simulink model "Project_SC"  (R2022a)
settings: Solver=FixedStepAuto  StartTime=0.0  StopTime=t_stop*5  FixedStep=t_step  EnableMultiTasking=on
values from neighbouring files (symbols this model uses):
  Ib = 1723*sqrt(2)    [analyticalStuff.m]
  J = p/2*Pb*M/(wmb^2)    (= 2380.03460376)    [analyticalStuff.m]
  p = 6    [analyticalStuff.m]
  Rr = 1.39e-3    (= 0.00139)    [analyticalStuff.m]
  Rs = 1.343e-3    (= 0.001343)    [analyticalStuff.m]
  Tb = 13.944e3    (= 13944)    [analyticalStuff.m]    (also in plotTorqueSpeedCurve.m)
  Tload = data.Tload    [plotTorqueSpeedCurve.m]    (also in torqueSpeedCurveData.mat = [-69720 -66874.2857143 -64028.5714286 -61182.8571429 -58337.)
  Vb = 331.98*sqrt(2)    [analyticalStuff.m]
  wb = 2*pi*fb    (= 314.159265359)    [analyticalStuff.m]
  we = 2*pi*fb    (= 314.159265359)    [analyticalStuff.m]
  Xlr = Llr*we    (= 0.0156451314149)    [analyticalStuff.m]
  Xls = Lls*we    (= 0.0327982273035)    [analyticalStuff.m]
  Xmstar = 1/(1/Xls+1/Xm+1/Xlr)    (= 0.0103944378454)    [analyticalStuff.m]
undefined symbols (not defined in the file or in its folder): fdr0, fds0, fqr0, fqs0, k, t_fault, wrotor_init
settings Model: Creator=kavita  LastModifiedBy=cakal
settings SolverCC: MaxConsecutiveZCs=1  ZeroCrossAlgorithm=Adaptive  AlgebraicLoopSolver=TrustRegion
settings DataIOCC: LimitDataPoints=on  SaveFormat=Array  SignalLoggingSaveFormat=ModelDataLogs  ReturnWorkspaceOutputs=off
settings OptimizationCC: ExpressionDepthLimit=2147483647  LifeSpan=inf
settings DebuggingCC: UnderspecifiedInitializationDetection=Classic  MergeDetectMultiDrivingBlocksExec=none  SolverPrmCheckMsg=warning  FcnCallInpInsideContextMsg=warning  UnconnectedInputMsg=warning  UnconnectedOutputMsg=warning  UnconnectedLineMsg=warning  StateNameClashWarn=warning  SFUnexpectedBacktrackingDiag=warning  SFNoUnconditionalDefaultTransitionDiag=warning  SFExecutionAtInitializationDiag=none  SFMachineParentedDataDiag=warning  ArithmeticOperatorsInVariantConditions=warning
settings HardwareCC: ProdBitPerPointer=32  ProdBitPerSizeT=32  ProdBitPerPtrDiffT=32  ProdLargestAtomicFloat=None  ProdIntDivRoundTo=Undefined  ProdEndianess=Unspecified  ProdWordSize=32  ProdHWDeviceType=32-bit Generic
settings ModelReferenceCC: PropagateSignalLabelsOutOfModel=off
settings SFSimCC: SimUseLocalCustomCode=off  CustomCodeUndefinedFunction=UseInterfaceOnly
settings RTWCC: RTWUseLocalCustomCode=off  DLArmComputeVersion=19.05
settings CodeAppCC: StateflowObjectComments=on
settings GRTTargetCC: TargetLangStandard=C89/C90 (ANSI)  CombineOutputUpdateFcns=off  GRTInterface=on
settings ConfigComp: CovMetricSettings=dw  CovSaveCumulativeToWorkspaceVar=on  CovSaveSingleToWorkspaceVar=on  CovExternalEMLEnable=off

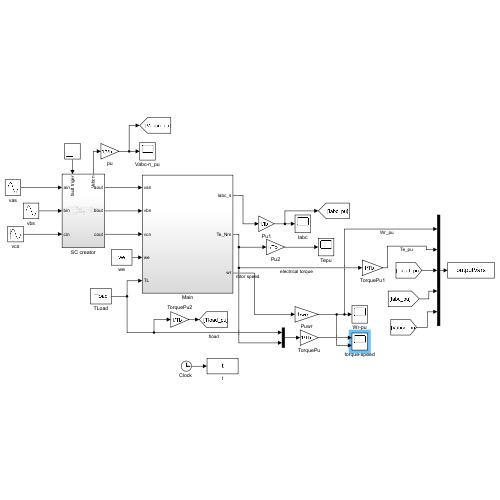
[thumbnail: Simulink's stored preview of the top-level diagram]
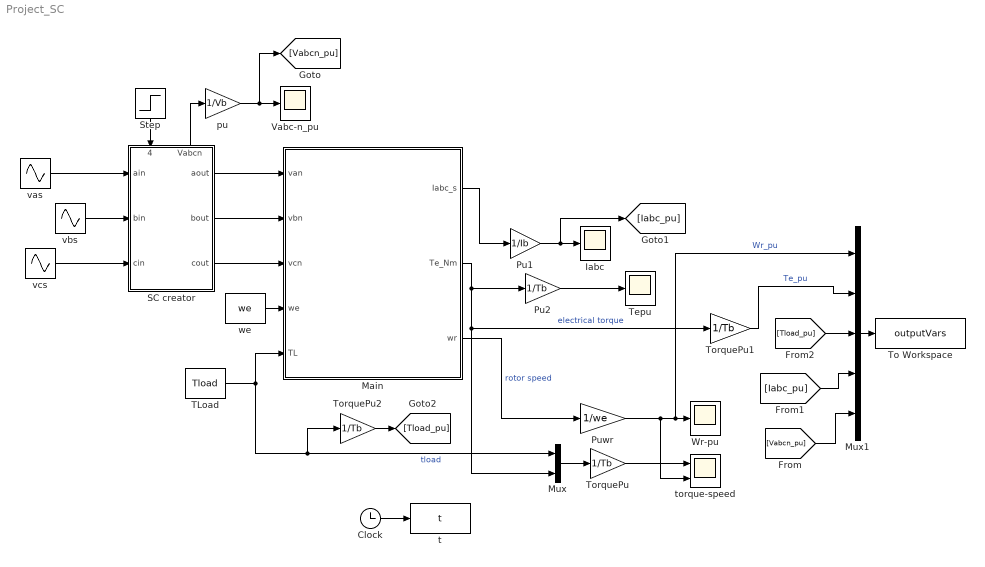
== system Project_SC ==
  "Clock " : Clock
  Iabc : Scope
  Main : Subsystem
  Mux : Mux  Inputs=2
  Mux1 : Mux  Inputs=5
  Pu1 : Gain  Gain=1/Ib
  Pu2 : Gain  Gain=1/Tb
  Puwr : Gain  Gain=1/we
  SC creator : Subsystem
      settings: PortSchema="{\"entries\":[{\"content\":{\"sides\":[{\"content\":{\"connectorIds\":[\"In1\",\"In2\",\"In3\"]},\"type\":\"ConnectorPlacement.EquallySpacedRectSide\",\"uuid\":\"9ddc0e81-d44d-497f-b86e-b421830f0102\"},{\"content\":{\"connectorIds\":[\"Out1\",\"Out2\",\"Out3\"],\"side\":\"RIGHT\"},\"type\":\"ConnectorPlacement.EquallySpacedRectSide\",\"uuid\":\"d203c1c5-ccdb-4337-8271-1be315a7d96e\"},{\"content\":{\"connectorIds\":[\"In4\",\"Out4\"],\"side\":\"TOP\"},\"type\":\"ConnectorPlacement.EquallySpacedRectSide\",\"uuid\":\"609a5643-1468-4543-bdb3-49e5cec14945\"}]},\"type\":\"ConnectorPlacement.EquallySpacedConnector\",\"uuid\":\"82ca2887-6272-42bf-b30c-e93039d72f15\"}],\"packageUris\":[\"http://schema.mathworks.com/mf0/Connector/R2020b\"],\"version\":\"1.0\"}"
  Step : Step  Time=t_fault(k)*0+2.5+1/50*90/360  Before=-1  SampleTime=0
  TLoad : Constant  Value=Tload
  Tepu : Scope
  To Workspace : ToWorkspace  VariableName=outputVars  SampleTime=-1
  TorquePu : Gain  Gain=1/Tb
  TorquePu1 : Gain  Gain=1/Tb
  TorquePu2 : Gain  Gain=1/Tb
  Vabc-n_pu : Scope
  Wr-pu : Scope
  pu : Gain  Gain=1/Vb
  t : ToWorkspace  VariableName=t  SampleTime=-1
  torque-speed : Scope  NumInputPorts=2
  vas : Sin  Amplitude=Vb  Frequency=wb  Phase=pi/2  SampleTime=0
  vbs : Sin  Amplitude=Vb  Frequency=wb  Phase=-120*pi/180+pi/2  SampleTime=0
  vcs : Sin  Amplitude=Vb  Frequency=wb  Phase=-240*pi/180+pi/2  SampleTime=0
  we : Constant  Value=we
  wires:
  we/1 -> Main/4(we)
  Main/2(Te_Nm) -> Pu2/1, TorquePu1/1, Mux/2  "electrical torque"
  Main/3(wr) -> Puwr/1  "rotor speed"
  "Clock "/1 -> t/1
  Mux/1 -> TorquePu/1
  TLoad/1 -> TorquePu2/1, Mux/1, Main/5(TL)  "tload"
  Main/1(Iabc_s) -> Pu1/1
  Pu1/1 -> [Iabc_pu], Iabc/1
  Pu2/1 -> Tepu/1
  Mux1/1 -> To Workspace/1
  Puwr/1 -> Mux1/1, Wr-pu/1, torque-speed/2  "Wr_pu"
  TorquePu1/1 -> Mux1/2  "Te_pu"
  vas/1 -> SC creator/1(ain)
  vbs/1 -> SC creator/2(bin)
  vcs/1 -> SC creator/3(cin)
  SC creator/1(aout) -> Main/1(van)
  SC creator/2(bout) -> Main/2(vbn)
  SC creator/3(cout) -> Main/3(vcn)
  Step/1 -> SC creator/4(fault triger)
  SC creator/4(Vabcn) -> pu/1
  pu/1 -> [Vabcn_pu], Vabc-n_pu/1
  [Vabcn_pu] -> Mux1/5
  [Iabc_pu] -> Mux1/4
  TorquePu/1 -> torque-speed/1
  [Tload_pu] -> Mux1/3
  TorquePu2/1 -> [Tload_pu]

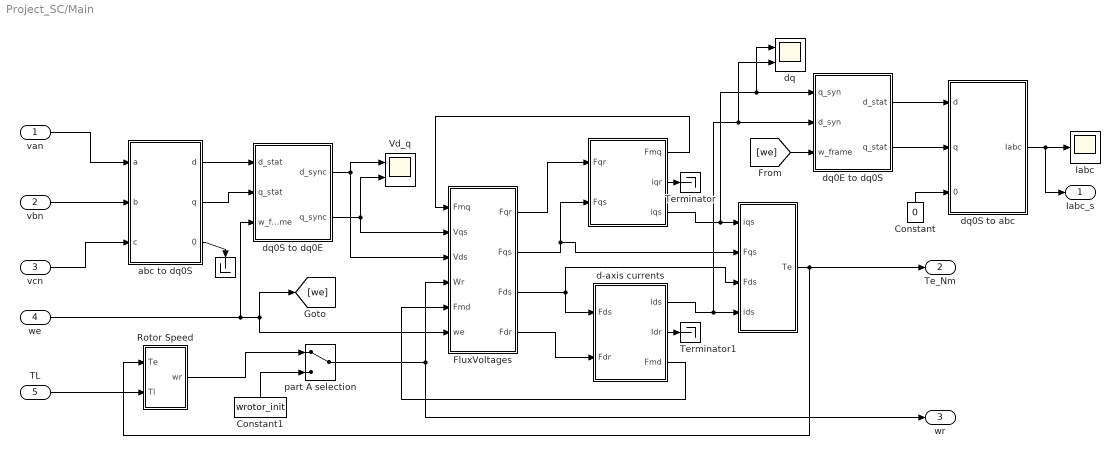
== system Project_SC/Main ==
  van : Inport
  vbn : Inport  Port=2
  vcn : Inport  Port=3
  we : Inport  Port=4
  TL : Inport  Port=5
  " " : Subsystem
  "  " : Subsystem
  "            " : Terminator
  Constant : Constant  Value=0
  Constant1 : Constant  Value=wrotor_init
  FluxVoltages : Subsystem
  Iabc : Scope
  Rotor Speed : Subsystem
  Terminator : Terminator
  Terminator1 : Terminator
  Vd_q : Scope  NumInputPorts=2
  abc to dq0S : Subsystem
  d-axis currents : Subsystem
  dq : Scope  NumInputPorts=2
  dq0E to dq0S : Subsystem
  dq0S to abc : Subsystem
  dq0S to dq0E : Subsystem
  part A selection : ManualSwitch
  Iabc_s : Outport  VectorParamsAs1DForOutWhenUnconnected=off
  Te_Nm : Outport  Port=2  VectorParamsAs1DForOutWhenUnconnected=off
  wr : Outport  Port=3  VectorParamsAs1DForOutWhenUnconnected=off
  wires:
  " "/1(Te) -> Te_Nm/1, Rotor Speed/1(Te)
  dq0S to dq0E/2(q_sync) -> Vd_q/2, FluxVoltages/2(Vqs)
  dq0S to dq0E/1(d_sync) -> Vd_q/1, FluxVoltages/3(Vds)
  abc to dq0S/3(0) -> "            "/1
  vbn/1 -> abc to dq0S/2(b)
  FluxVoltages/2(Fqs) -> " "/2(Fqs), "  "/2(Fqs)
  FluxVoltages/4(Fdr) -> d-axis currents/2(Fdr)
  FluxVoltages/1(Fqr) -> "  "/1(Fqr)
  FluxVoltages/3(Fds) -> " "/3(Fds), d-axis currents/1(Fds)
  vcn/1 -> abc to dq0S/3(c)
  TL/1 -> Rotor Speed/2(Tl)
  "  "/1(Fmq) -> FluxVoltages/1(Fmq)
  part A selection/1 -> wr/1, FluxVoltages/4(Wr)
  d-axis currents/2(Idr) -> Terminator1/1
  d-axis currents/1(ids) -> dq0E to dq0S/2(d_syn), dq/2, " "/4(ids)
  d-axis currents/3(Fmd) -> FluxVoltages/5(Fmd)
  "  "/2(iqr) -> Terminator/1
  "  "/3(iqs) -> dq/1, dq0E to dq0S/1(q_syn), " "/1(iqs)
  van/1 -> abc to dq0S/1(a)
  abc to dq0S/1(d) -> dq0S to dq0E/1(d_stat)
  abc to dq0S/2(q) -> dq0S to dq0E/2(q_stat)
  we/1 -> dq0S to dq0E/3(w_frame), [we], FluxVoltages/6(we)
  [we] -> dq0E to dq0S/3(w_frame)
  dq0E to dq0S/2(q_stat) -> dq0S to abc/2(q)
  dq0E to dq0S/1(d_stat) -> dq0S to abc/1(d)
  Constant/1 -> dq0S to abc/3(0)
  dq0S to abc/1(Iabc) -> Iabc/1, Iabc_s/1
  Rotor Speed/1(wr) -> part A selection/1
  Constant1/1 -> part A selection/2

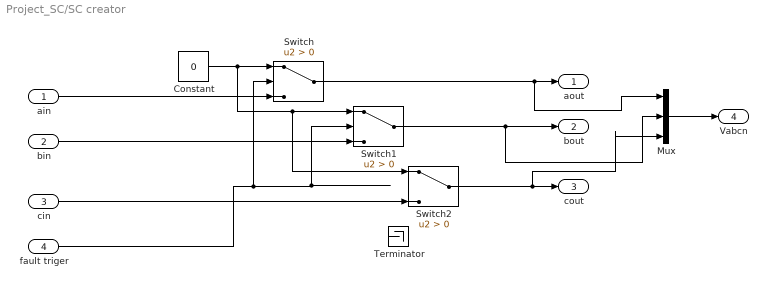
== system Project_SC/SC creator ==
  ain : Inport
  bin : Inport  Port=2
  cin : Inport  Port=3
  fault triger : Inport  Port=4
  Constant : Constant  Value=0
  Mux : Mux  Inputs=3
  Switch : Switch  Criteria=u2 > Threshold  SaturateOnIntegerOverflow=off  InputSameDT=off
  Switch1 : Switch  Criteria=u2 > Threshold  SaturateOnIntegerOverflow=off  InputSameDT=off
  Switch2 : Switch  Criteria=u2 > Threshold  SaturateOnIntegerOverflow=off  InputSameDT=off
  Terminator : Terminator
  aout : Outport
  bout : Outport  Port=2
  cout : Outport  Port=3
  Vabcn : Outport  Port=4
  wires:
  Constant/1 -> Switch/1, Switch1/1, Switch2/1
  bin/1 -> Switch1/3
  ain/1 -> Switch/3
  cin/1 -> Switch2/3
  fault triger/1 -> Switch/2, Switch1/2
  Switch/1 -> Mux/1, aout/1
  Mux/1 -> Vabcn/1
  Switch1/1 -> Mux/2, bout/1
  Switch2/1 -> Mux/3, cout/1

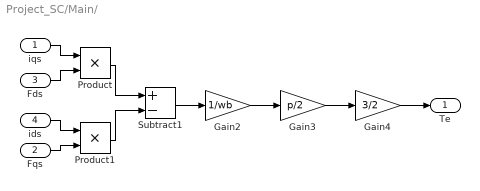
== system Project_SC/Main/  ==
  iqs : Inport
  Fqs : Inport  Port=2
  Fds : Inport  Port=3
  ids : Inport  Port=4
  Gain2 : Gain  Gain=1/wb
  Gain3 : Gain  Gain=p/2
  Gain4 : Gain  Gain=3/2
  Product : Product  RndMeth=Zero
  Product1 : Product  RndMeth=Zero
  Subtract1 : Sum  Inputs=+-
  Te : Outport  VectorParamsAs1DForOutWhenUnconnected=off
  wires:
  Gain4/1 -> Te/1
  Gain3/1 -> Gain4/1
  Gain2/1 -> Gain3/1
  Subtract1/1 -> Gain2/1
  Product1/1 -> Subtract1/2
  Product/1 -> Subtract1/1
  Fqs/1 -> Product1/2
  ids/1 -> Product1/1
  Fds/1 -> Product/2
  iqs/1 -> Product/1

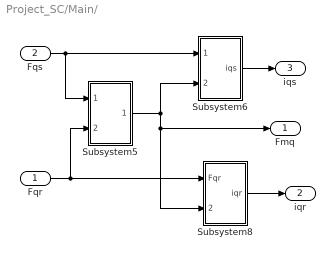
== system Project_SC/Main/   ==
  Fqr : Inport
  Fqs : Inport  Port=2
  Subsystem5 : Subsystem
  Subsystem6 : Subsystem
  Subsystem8 : Subsystem
  Fmq : Outport  VectorParamsAs1DForOutWhenUnconnected=off
  iqr : Outport  Port=2  VectorParamsAs1DForOutWhenUnconnected=off
  iqs : Outport  Port=3  VectorParamsAs1DForOutWhenUnconnected=off
  wires:
  Subsystem5/1(Fmq) -> Subsystem8/2(Fmq), Fmq/1, Subsystem6/2(Fmq)
  Fqs/1 -> Subsystem6/1(Fqs), Subsystem5/1(Fqs)
  Fqr/1 -> Subsystem8/1(Fqr), Subsystem5/2(Fqr)
  Subsystem6/1(iqs) -> iqs/1
  Subsystem8/1(iqr) -> iqr/1

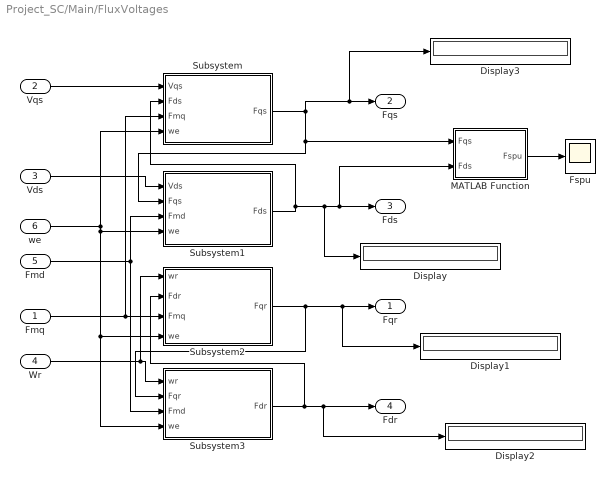
== system Project_SC/Main/FluxVoltages ==
  Fmq : Inport
  Vqs : Inport  Port=2
  Vds : Inport  Port=3
  Wr : Inport  Port=4
  Fmd : Inport  Port=5
  we : Inport  Port=6
  Display{,1..3} (4 alike) : Display
      settings: Decimation=6
  Fspu : Scope
  MATLAB Function : MATLAB Function  TreatAsAtomicUnit=on
  Subsystem : Subsystem
  Subsystem1 : Subsystem
  Subsystem2 : Subsystem
  Subsystem3 : Subsystem
  Fqr : Outport  VectorParamsAs1DForOutWhenUnconnected=off
  Fqs : Outport  Port=2  VectorParamsAs1DForOutWhenUnconnected=off
  Fds : Outport  Port=3  VectorParamsAs1DForOutWhenUnconnected=off
  Fdr : Outport  Port=4  VectorParamsAs1DForOutWhenUnconnected=off
  wires:
  Subsystem3/1(Fdr) -> Display2/1, Fdr/1, Subsystem2/2(Fdr)
  Subsystem2/1(Fqr) -> Subsystem3/2(Fqr), Display1/1, Fqr/1
  Subsystem/1(Fqs) -> Display3/1, Fqs/1, MATLAB Function/1(Fqs), Subsystem1/2(Fqs)
  Subsystem1/1(Fds) -> Subsystem/2(Fds), Display/1, MATLAB Function/2(Fds), Fds/1
  Vqs/1 -> Subsystem/1(Vqs)
  Vds/1 -> Subsystem1/1(Vds)
  Fmd/1 -> Subsystem1/3(Fmd), Subsystem3/3(Fmd)
  Fmq/1 -> Subsystem2/3(Fmq), Subsystem/3(Fmq)
  Wr/1 -> Subsystem3/1(wr), Subsystem2/1(wr)
  we/1 -> Subsystem1/4(we), Subsystem3/4(we), Subsystem2/4(we), Subsystem/4(we)
  MATLAB Function/1(Fspu) -> Fspu/1

== system Project_SC/Main/Rotor Speed ==
  Te : Inport
  Tl : Inport  Port=2
  Gain1 : Gain  Gain=1/J
  Gain2 : Gain  Gain=p/2
  Integrator : Integrator  InitialCondition=wrotor_init
  Subtract : Sum  Inputs=+-
  wr : Outport  VectorParamsAs1DForOutWhenUnconnected=off
  wires:
  Te/1 -> Subtract/1
  Gain1/1 -> Gain2/1
  Subtract/1 -> Gain1/1
  Gain2/1 -> Integrator/1
  Integrator/1 -> wr/1
  Tl/1 -> Subtract/2

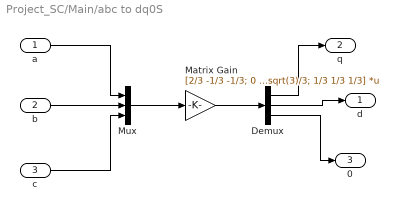
== system Project_SC/Main/abc to dq0S ==
  a : Inport
  b : Inport  Port=2
  c : Inport  Port=3
  Demux : Demux  Outputs=3
  Matrix Gain : Gain  Gain=[2/3 -1/3 -1/3; 0 -sqrt(3)/3 sqrt(3)/3; 1/3 1/3 1/3]  Multiplication=Matrix(K*u)  SaturateOnIntegerOverflow=on  OutDataTypeStr=Inherit: Same as input  ParamDataTypeStr=Inherit: Same as input
  Mux : Mux  Inputs=3
  d : Outport  VectorParamsAs1DForOutWhenUnconnected=off
  q : Outport  Port=2  VectorParamsAs1DForOutWhenUnconnected=off
  0 : Outport  Port=3  VectorParamsAs1DForOutWhenUnconnected=off
  wires:
  a/1 -> Mux/1
  b/1 -> Mux/2
  c/1 -> Mux/3
  Demux/1 -> q/1
  Demux/2 -> d/1
  Demux/3 -> 0/1
  Mux/1 -> Matrix Gain/1
  Matrix Gain/1 -> Demux/1

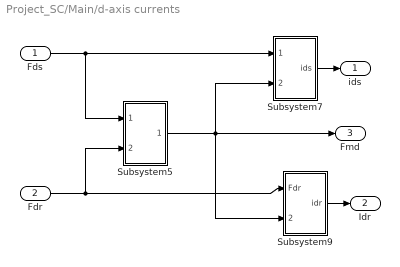
== system Project_SC/Main/d-axis currents ==
  Fds : Inport
  Fdr : Inport  Port=2
  Subsystem5 : Subsystem
  Subsystem7 : Subsystem
  Subsystem9 : Subsystem
  ids : Outport  VectorParamsAs1DForOutWhenUnconnected=off
  Idr : Outport  Port=2  VectorParamsAs1DForOutWhenUnconnected=off
  Fmd : Outport  Port=3  VectorParamsAs1DForOutWhenUnconnected=off
  wires:
  Subsystem5/1(Fmd) -> Subsystem7/2(Fmd), Subsystem9/2(Fmd), Fmd/1
  Fds/1 -> Subsystem7/1(Fds), Subsystem5/1(Fds)
  Fdr/1 -> Subsystem9/1(Fdr), Subsystem5/2(Fdr)
  Subsystem7/1(ids) -> ids/1
  Subsystem9/1(idr) -> Idr/1

== system Project_SC/Main/dq0E to dq0S ==
  q_syn : Inport
  d_syn : Inport  Port=2
  w_frame : Inport  Port=3
  Clock : Clock
  MATLAB Function : MATLAB Function  TreatAsAtomicUnit=on
  d_stat : Outport  VectorParamsAs1DForOutWhenUnconnected=off
  q_stat : Outport  Port=2  VectorParamsAs1DForOutWhenUnconnected=off
  wires:
  q_syn/1 -> MATLAB Function/1(Vq_syn)
  d_syn/1 -> MATLAB Function/2(Vd_syn)
  MATLAB Function/2(Vd_stat) -> d_stat/1
  MATLAB Function/1(Vq_stat) -> q_stat/1
  w_frame/1 -> MATLAB Function/4(w_frame)
  Clock/1 -> MATLAB Function/3(time)

== system Project_SC/Main/dq0S to abc ==
  d : Inport
  q : Inport  Port=2
  0 : Inport  Port=3
  Matrix Gain : Gain  Gain=[1 0 1; -1/2 -sqrt(3)/2 1; -1/2 sqrt(3)/2 1]  Multiplication=Matrix(K*u)  SaturateOnIntegerOverflow=on  OutDataTypeStr=Inherit: Same as input  ParamDataTypeStr=Inherit: Same as input
  Mux : Mux  Inputs=3
  Iabc : Outport  VectorParamsAs1DForOutWhenUnconnected=off
  wires:
  d/1 -> Mux/2
  q/1 -> Mux/1
  0/1 -> Mux/3
  Matrix Gain/1 -> Iabc/1
  Mux/1 -> Matrix Gain/1

== system Project_SC/Main/dq0S to dq0E ==
  d_stat : Inport
  q_stat : Inport  Port=2
  w_frame : Inport  Port=3
  Clock : Clock
  MATLAB Function : MATLAB Function  TreatAsAtomicUnit=on
  d_sync : Outport  VectorParamsAs1DForOutWhenUnconnected=off
  q_sync : Outport  Port=2  VectorParamsAs1DForOutWhenUnconnected=off
  wires:
  d_stat/1 -> MATLAB Function/1(d_stat)
  q_stat/1 -> MATLAB Function/2(q_stat)
  MATLAB Function/2(Vd_syn) -> d_sync/1
  MATLAB Function/1(Vq_syn) -> q_sync/1
  w_frame/1 -> MATLAB Function/4(w_frame)
  Clock/1 -> MATLAB Function/3(time)

== system Project_SC/Main/  /Subsystem5 ==
  Fqs : Inport
  Fqr : Inport  Port=2
  Fqr/Xlr : Gain  Gain=1/Xlr
  Fqs/Xls : Gain  Gain=1/Xls
  Gain : Gain  Gain=Xmstar
  Sum : Sum
  Fmq : Outport  VectorParamsAs1DForOutWhenUnconnected=off
  wires:
  Gain/1 -> Fmq/1
  Sum/1 -> Gain/1
  Fqr/1 -> Fqr/Xlr/1
  Fqs/1 -> Fqs/Xls/1
  Fqs/Xls/1 -> Sum/1
  Fqr/Xlr/1 -> Sum/2

== system Project_SC/Main/  /Subsystem6 ==
  Fqs : Inport
  Fmq : Inport  Port=2
  Gain : Gain  Gain=1/Xls
  Subtract : Sum  Inputs=+-
  iqs : Outport  VectorParamsAs1DForOutWhenUnconnected=off
  wires:
  Gain/1 -> iqs/1
  Subtract/1 -> Gain/1
  Fmq/1 -> Subtract/2
  Fqs/1 -> Subtract/1

== system Project_SC/Main/  /Subsystem8 ==
  Fqr : Inport
  Fmq : Inport  Port=2
  Gain : Gain  Gain=1/Xlr
  Subtract : Sum  Inputs=+-
  iqr : Outport  VectorParamsAs1DForOutWhenUnconnected=off
  wires:
  Subtract/1 -> Gain/1
  Fqr/1 -> Subtract/1
  Fmq/1 -> Subtract/2
  Gain/1 -> iqr/1

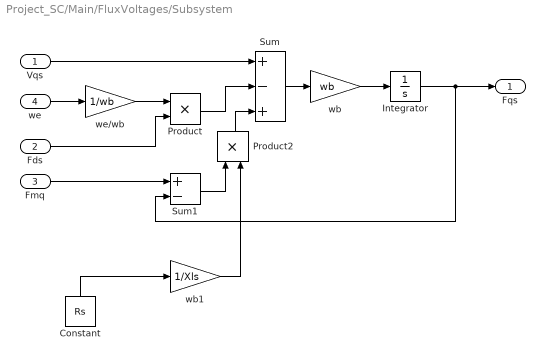
== system Project_SC/Main/FluxVoltages/Subsystem ==
  Vqs : Inport
  Fds : Inport  Port=2
  Fmq : Inport  Port=3
  we : Inport  Port=4
  Constant : Constant  Value=Rs
  Integrator : Integrator  InitialCondition=fqs0
  Product : Product  RndMeth=Zero
  Product2 : Product  RndMeth=Zero
  Sum : Sum  Inputs=+-+
  Sum1 : Sum  Inputs=+-
  wb : Gain  Gain=wb
  wb1 : Gain  Gain=1/Xls
  we/wb : Gain  Gain=1/wb
  Fqs : Outport  VectorParamsAs1DForOutWhenUnconnected=off
  wires:
  Vqs/1 -> Sum/1
  we/1 -> we/wb/1
  we/wb/1 -> Product/1
  Fds/1 -> Product/2
  Product/1 -> Sum/2
  Sum/1 -> wb/1
  wb/1 -> Integrator/1
  Product2/1 -> Sum/3
  Sum1/1 -> Product2/1
  Fmq/1 -> Sum1/1
  Integrator/1 -> Sum1/2, Fqs/1
  Constant/1 -> wb1/1
  wb1/1 -> Product2/2

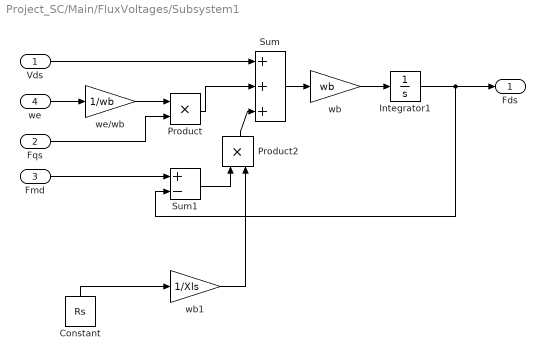
== system Project_SC/Main/FluxVoltages/Subsystem1 ==
  Vds : Inport
  Fqs : Inport  Port=2
  Fmd : Inport  Port=3
  we : Inport  Port=4
  Constant : Constant  Value=Rs
  Integrator1 : Integrator  InitialCondition=fds0
  Product : Product  RndMeth=Zero
  Product2 : Product  RndMeth=Zero
  Sum : Sum  Inputs=+++
  Sum1 : Sum  Inputs=+-
  wb : Gain  Gain=wb
  wb1 : Gain  Gain=1/Xls
  we/wb : Gain  Gain=1/wb
  Fds : Outport  VectorParamsAs1DForOutWhenUnconnected=off
  wires:
  Product2/1 -> Sum/3
  wb/1 -> Integrator1/1
  Sum/1 -> wb/1
  Product/1 -> Sum/2
  Fqs/1 -> Product/2
  we/wb/1 -> Product/1
  we/1 -> we/wb/1
  Vds/1 -> Sum/1
  Fmd/1 -> Sum1/1
  Integrator1/1 -> Sum1/2, Fds/1
  Constant/1 -> wb1/1
  Sum1/1 -> Product2/1
  wb1/1 -> Product2/2

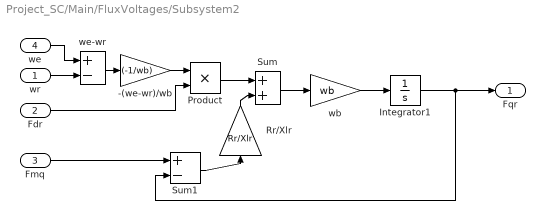
== system Project_SC/Main/FluxVoltages/Subsystem2 ==
  wr : Inport
  Fdr : Inport  Port=2
  Fmq : Inport  Port=3
  we : Inport  Port=4
  -(we-wr)/wb : Gain  Gain=(-1/wb)
  Integrator1 : Integrator  InitialCondition=fqr0
  Product : Product  RndMeth=Zero
  Rr/Xlr : Gain  Gain=Rr/Xlr
  Sum : Sum
  Sum1 : Sum  Inputs=+-
  wb : Gain  Gain=wb
  we-wr : Sum  Inputs=+-
  Fqr : Outport  VectorParamsAs1DForOutWhenUnconnected=off
  wires:
  Sum/1 -> wb/1
  wb/1 -> Integrator1/1
  Sum1/1 -> Rr/Xlr/1
  Rr/Xlr/1 -> Sum/2
  Product/1 -> Sum/1
  Fdr/1 -> Product/2
  -(we-wr)/wb/1 -> Product/1
  we-wr/1 -> -(we-wr)/wb/1
  we/1 -> we-wr/1
  wr/1 -> we-wr/2
  Fmq/1 -> Sum1/1
  Integrator1/1 -> Sum1/2, Fqr/1

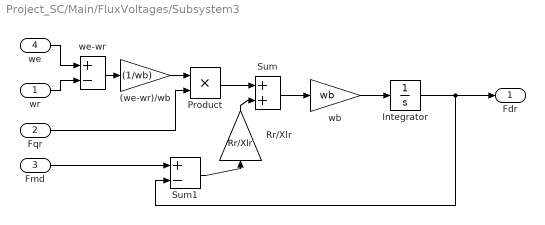
== system Project_SC/Main/FluxVoltages/Subsystem3 ==
  wr : Inport
  Fqr : Inport  Port=2
  Fmd : Inport  Port=3
  we : Inport  Port=4
  (we-wr)/wb : Gain  Gain=(1/wb)
  Integrator : Integrator  InitialCondition=fdr0
  Product : Product  RndMeth=Zero
  Rr/Xlr : Gain  Gain=Rr/Xlr
  Sum : Sum
  Sum1 : Sum  Inputs=+-
  wb : Gain  Gain=wb
  we-wr : Sum  Inputs=+-
  Fdr : Outport  VectorParamsAs1DForOutWhenUnconnected=off
  wires:
  wr/1 -> we-wr/2
  we/1 -> we-wr/1
  we-wr/1 -> (we-wr)/wb/1
  (we-wr)/wb/1 -> Product/1
  Fqr/1 -> Product/2
  Product/1 -> Sum/1
  Rr/Xlr/1 -> Sum/2
  Sum1/1 -> Rr/Xlr/1
  wb/1 -> Integrator/1
  Sum/1 -> wb/1
  Fmd/1 -> Sum1/1
  Integrator/1 -> Sum1/2, Fdr/1

== system Project_SC/Main/d-axis currents/Subsystem5 ==
  Fds : Inport
  Fdr : Inport  Port=2
  Fdr/Xlr : Gain  Gain=1/Xlr
  Fds/Xls : Gain  Gain=1/Xls
  Gain : Gain  Gain=Xmstar
  Sum : Sum
  Fmd : Outport  VectorParamsAs1DForOutWhenUnconnected=off
  wires:
  Gain/1 -> Fmd/1
  Sum/1 -> Gain/1
  Fdr/1 -> Fdr/Xlr/1
  Fds/1 -> Fds/Xls/1
  Fds/Xls/1 -> Sum/1
  Fdr/Xlr/1 -> Sum/2

== system Project_SC/Main/d-axis currents/Subsystem7 ==
  Fds : Inport
  Fmd : Inport  Port=2
  Gain : Gain  Gain=1/Xls
  Subtract : Sum  Inputs=+-
  ids : Outport  VectorParamsAs1DForOutWhenUnconnected=off
  wires:
  Subtract/1 -> Gain/1
  Fds/1 -> Subtract/1
  Fmd/1 -> Subtract/2
  Gain/1 -> ids/1

== system Project_SC/Main/d-axis currents/Subsystem9 ==
  Fdr : Inport
  Fmd : Inport  Port=2
  Gain : Gain  Gain=1/Xlr
  Subtract : Sum  Inputs=+-
  idr : Outport  VectorParamsAs1DForOutWhenUnconnected=off
  wires:
  Subtract/1 -> Gain/1
  Fdr/1 -> Subtract/1
  Fmd/1 -> Subtract/2
  Gain/1 -> idr/1

== matlab function Project_SC/Main/dq0S to dq0E/MATLAB Function ==
  data: d_stat input; q_stat input; Vq_syn output; time input; w_frame input; Vd_syn output
function [Vq_syn,Vd_syn] = fcn(d_stat,q_stat,time,w_frame)


Vdq_s_comp = q_stat - 1i*d_stat;
Vdq_e_comp = Vdq_s_comp * exp(-1i*w_frame*time);
Vq_syn = real(Vdq_e_comp);
Vd_syn = -imag(Vdq_e_comp);

== matlab function Project_SC/Main/dq0E to dq0S/MATLAB Function ==
  data: Vq_syn input; Vd_syn input; Vq_stat output; time input; w_frame input; Vd_stat output
function [Vq_stat,Vd_stat] = fcn(Vq_syn,Vd_syn,time,w_frame)


Vdq_e_comp = Vq_syn - 1i*Vd_syn;
Vdq_s_comp = Vdq_e_comp * exp(1i*w_frame*time);
Vq_stat = real(Vdq_s_comp);
Vd_stat = -imag(Vdq_s_comp);

== matlab function Project_SC/Main/FluxVoltages/MATLAB Function ==
  data: Fqs input; Fspu output; Fds input
function Fspu = fcn(Fqs,Fds)

Vb = 376;
Fspu = sqrt(Fqs^2+Fds^2)/Vb;
